simulink model "HQEV_MiL_20160830_integrate_r2017a"  (Simulink 8.9)
settings: Solver=FixedStepDiscrete  StartTime=0.0  StopTime=inf  FixedStep=0.01  RelTol=1e-3  EnableMultiTasking=on
PostLoadFcn:
  | , if any(exist('dsrtsu_mdlpostloadfcn', 'file') == [2, 3, 6]), try dsrtsu_mdlpostloadfcn('Execute', bdroot); catch fprintf('Error in PostLoadFcn (dsrtsu_mdlpostloadfcn) for model "%s":\n %s\n', bdroot, lasterr); end, end,
values from neighbouring files (symbols this model uses):
  Bat_C_Ah = 36    [parameter_V1.mat]
  Bat_ocv_xIndex = [5 10 20 30 40 50 60 70 80 90 95]    [parameter_V1.mat]
  Bat_ocv_z = [329 332 340 345 347 351 358 372 377 386 391]    [parameter_V1.mat]
  Bat_R_ohm_z = [4.41 3.46 1.57 1.07 0.76 0.63 0.55 0.44 0.41 0.4 0.4 3.14 ... (66 elements, 11x6)]    [parameter_V1.mat]
  Bat_SOC_Init = 90    [parameter_V1.mat]
  Env_hum_pct_Ambient = 30    [parameter_V1.mat]
  Env_Slope_deg = 0    [parameter_V1.mat]
  Env_Temp_degC_Ambient = 25    [parameter_V1.mat]
  Env_v_kmph_HWind = 0    [parameter_V1.mat]
  Reducer_F_i = 7.23    [parameter_V1.mat]
  Reducer_R_i = 7.23    [parameter_V1.mat]
  Veh =     [parameter_V1.mat]
  Veh_A_m2_Fr = 2.246    [parameter_V1.mat]
  Veh_F_Brake =     [parameter_V1.mat]
  Veh_fac_AirDrag = 0.326    [parameter_V1.mat]
  Veh_fac_WhDragFrict_0 = 0.011    [parameter_V1.mat]
  Veh_g_mps2_C = 9.81    [parameter_V1.mat]
  Veh_GainBrake =     [parameter_V1.mat]
  Veh_h_m_COGHigh = 0.5    [parameter_V1.mat]
  Veh_J_kgm2_Wh = 1.3635    [parameter_V1.mat]
  Veh_L_m_AxlBas = 2.63    [parameter_V1.mat]
  Veh_M_kg = 1427    [parameter_V1.mat]
  Veh_mu_Brake = 0.4    [parameter_V1.mat]
  Veh_mu_Tyre =     [parameter_V1.mat]
  Veh_num_FrictPair = 8    [parameter_V1.mat]
  Veh_pct_Brk = 70    [parameter_V1.mat]
  Veh_r_dyn =     [parameter_V1.mat]
  Veh_r_m_BrkDisk = 0.136    [parameter_V1.mat]
  Veh_rho_kgpm3_Air = 1.2258    [parameter_V1.mat]
undefined symbols (not defined in the file or in its folder): DiscIntNeverNeededParam, p_bool_False_M, p_bool_True_M
libraries: BaseOperationLib_Browser x38, simulink x8, DTQC_lib x1, ERR_lib x1, MQM_lib x1, PTCL_lib x1, PUD_lib x1, TQD_lib x1, TQR_lib x1, VMM_lib x1, ACCA_lib x1, BBCA_lib x1
(part 7 of 15)

== system HQEV_MiL_20160830_integrate_r2017a/MiL/Test_Integration/MCU_FF/MCU/MCU ==
  In1 : Inport
  Bus Selector : BusSelector  OutputSignals=HCU.HCU_SleepIndication,BMS.BMS_MainPlusContactorCoilState,BMS.BMS_MainMinusContactorCoilState,HCU.HCU_StatusTMRequestToMCU1,HCU.HCU_StopRequestToMCU1,BMS.BMS_PrechargeContactorCoilState,HCU.HCU_RapidDischargeCmdToMCU1,Motor_F.EM1_U,Charger.Charger_OutputVoltage
  Chart : Stateflow chart  TreatAsAtomicUnit=on
  GSD : Subsystem  TreatAsAtomicUnit=on
  Init : Subsystem  TreatAsAtomicUnit=on
  Invalid : Subsystem  TreatAsAtomicUnit=on
  Multiport Switch : MultiPortSwitch  DataPortOrder=Zero-based contiguous  Inputs=9  zeroidx=on
  Precharge : Subsystem  TreatAsAtomicUnit=on
  Rapid_Discharge : Subsystem  TreatAsAtomicUnit=on
  Sleep : Subsystem  TreatAsAtomicUnit=on
  Standby : Subsystem  TreatAsAtomicUnit=on
  Stop : Subsystem  TreatAsAtomicUnit=on
  Torque_Control : Subsystem  TreatAsAtomicUnit=on
  out : Outport
  wires:
  Chart/2(Sleep_Act()) -> [Sleep_Act]
  Chart/3(Init_Act()) -> [Init_Act]
  Chart/4(Precharge_Act()) -> [Precharge_Act]
  Chart/5(Standby_Act()) -> [Standby_Act]
  Chart/6(Torque_Control_Act()) -> [Torque_Control_Act]
  Chart/7(Stop_Act()) -> [Stop_Act]
  Chart/8(GSD_Act()) -> [GSD_Act]
  Chart/9(Rapid_Discharge_Act()) -> [Rapid_Discharge_Act]
  Chart/10(Invalid_Act()) -> [Invalid_Act]
  Chart/1(MCU1_TMStatus) -> [MCU1_TMStatus]
  [Init_Act] -> Init/Trigger
  [Precharge_Act] -> Precharge/Trigger
  [Torque_Control_Act] -> Torque_Control/Trigger
  [Stop_Act] -> Stop/Trigger
  [Rapid_Discharge_Act] -> Rapid_Discharge/Trigger
  [Invalid_Act] -> Invalid/Trigger
  [Standby_Act] -> Standby/Trigger
  [GSD_Act] -> GSD/Trigger
  Init/1(Out1) -> Multiport Switch/2
  Precharge/1(Out1) -> Multiport Switch/3
  Standby/1(Out1) -> Multiport Switch/4
  Torque_Control/1(Out1) -> Multiport Switch/5
  Stop/1(Out1) -> Multiport Switch/6
  GSD/1(Out1) -> Multiport Switch/7
  Rapid_Discharge/1(Out1) -> Multiport Switch/8
  Invalid/1(Out1) -> Multiport Switch/9
  [Sleep_Act] -> Sleep/Trigger
  Sleep/1(Out1) -> Multiport Switch/10
  [MCU1_TMStatus] -> Multiport Switch/1
  In1/1 -> Init/1(In1), Precharge/1(In1), Standby/1(In1), Torque_Control/1(In1), Stop/1(In1), GSD/1(In1), Rapid_Discharge/1(In1), Invalid/1(In1), Sleep/1(In1), Bus Selector/1
  Multiport Switch/1 -> out/1
  Bus Selector/1 -> Chart/1(SleepInd)  "<HCU_SleepIndication>"
  Bus Selector/2 -> Chart/2(BMS_MainPlusContactorState)  "<BMS_MainPlusContactorCoilState>"
  Bus Selector/3 -> Chart/3(BMS_MainMinusContactorCoilState)  "<BMS_MainMinusContactorCoilState>"
  Bus Selector/4 -> Chart/4(HCU_StatusTMRequestToMCU1)  "<HCU_StatusTMRequestToMCU1>"
  Bus Selector/5 -> Chart/5(HCU_StopRequestToMCU1)  "<HCU_StopRequestToMCU1>"
  Bus Selector/6 -> Chart/6(BMS_PrechargeContactorCoilState)  "<BMS_PrechargeContactorCoilState>"
  Bus Selector/7 -> Chart/7(HCU_RapidDischargeCmdToMCU1)  "<HCU_RapidDischargeCmdToMCU1>"
  Bus Selector/8 -> Chart/8(Uc1)  "<EM1_U>"
  Bus Selector/9 -> Chart/9(Charger_OutputVoltage)  "<Charger_OutputVoltage>"

== system HQEV_MiL_20160830_integrate_r2017a/MiL/Test_Integration/MCU_FF/MCU/Signal ==
  bus : Inport
  Bus Creator1 : BusCreator  Inputs=17
  Checksum_MCU1_1 : Subsystem
  Checksum_MCU1_2 : Subsystem
  LiveCounter_MCU1_1 : Subsystem
  LiveCounter_MCU1_2 : Subsystem
  MCU1_ActTMTorque : Subsystem
  MCU1_ActualTMTorqueValid : Subsystem
  MCU1_CalTMTorque : Subsystem
  MCU1_CoolingRequest : Subsystem
  MCU1_PrechargeAllow : Subsystem
  MCU1_ShutdownEnable : Subsystem
  MCU1_TMCapacitanceVoltage : Subsystem
  MCU1_TMErrorStatus : Subsystem
  MCU1_TMSpeed : Subsystem
  MCU1_TMStatus : Subsystem
  MCU1_TM_MAGTorque : Subsystem
  MCU1_TM_MAMTorque : Subsystem
  MCU1_trq_req : Subsystem
  Out1 : Outport
  wires:
  Checksum_MCU1_1/1(out) -> Bus Creator1/1  "Checksum_MCU1_1"
  MCU1_TMSpeed/1(out) -> Bus Creator1/2  "MCU1_TMSpeed"
  MCU1_ActTMTorque/1(out) -> Bus Creator1/3  "MCU1_ActTMTorque"
  LiveCounter_MCU1_1/1(out) -> Bus Creator1/4  "LiveCounter_MCU1_1"
  MCU1_TMCapacitanceVoltage/1(out) -> Bus Creator1/5  "MCU1_TMCapacitanceVoltage"
  MCU1_ActualTMTorqueValid/1(out) -> Bus Creator1/6  "MCU1_ActualTMTorqueValid"
  MCU1_PrechargeAllow/1(out) -> Bus Creator1/7  "MCU1_PrechargeAllow"
  MCU1_TMStatus/1(out) -> Bus Creator1/8  "MCU1_TMStatus"
  MCU1_TMErrorStatus/1(out) -> Bus Creator1/9  "MCU1_TMErrorStatus"
  Checksum_MCU1_2/1(out) -> Bus Creator1/10  "Checksum_MCU1_2"
  MCU1_TM_MAMTorque/1(out) -> Bus Creator1/11  "MCU1_TM_MAMTorque"
  MCU1_TM_MAGTorque/1(out) -> Bus Creator1/12  "MCU1_TM_MAGTorque"
  LiveCounter_MCU1_2/1(out) -> Bus Creator1/13  "LiveCounter_MCU1_2"
  MCU1_CalTMTorque/1(out) -> Bus Creator1/14  "MCU1_CalTMTorque"
  MCU1_CoolingRequest/1(out) -> Bus Creator1/15  "MCU1_CoolingRequest"
  MCU1_trq_req/1(out) -> Bus Creator1/16  "MCU1_trq_req"
  bus/1 -> Checksum_MCU1_1/1(In1), MCU1_TMSpeed/1(In1), MCU1_ActTMTorque/1(In1), LiveCounter_MCU1_1/1(In1), MCU1_TMCapacitanceVoltage/1(In1), MCU1_ActualTMTorqueValid/1(In1), MCU1_PrechargeAllow/1(In1), MCU1_TMStatus/1(In1), MCU1_TMErrorStatus/1(In1), Checksum_MCU1_2/1(In1), MCU1_TM_MAMTorque/1(In1), MCU1_TM_MAGTorque/1(In1), LiveCounter_MCU1_2/1(In1), MCU1_CalTMTorque/1(In1), MCU1_CoolingRequest/1(In1), MCU1_ShutdownEnable/1(In1), MCU1_trq_req/1(In1)
  Bus Creator1/1 -> Out1/1
  MCU1_ShutdownEnable/1(out) -> Bus Creator1/17  "MCU1_ShutdownEnable"

== system HQEV_MiL_20160830_integrate_r2017a/MiL/Test_Integration/MCU_RR/MCU/MCU ==
  In1 : Inport
  Bus Creator : BusCreator  Inputs=14
  Subsystem14 : Subsystem
  Out1 : Outport
  wires:
  In1/1 -> Subsystem14/1(In1)
  Subsystem14/1(MCU2_TMSpeed) -> Bus Creator/1  "MCU2_TMSpeed"
  Subsystem14/2(MCU2_ActTMTorque) -> Bus Creator/2  "MCU2_ActTMTorque"
  Subsystem14/3(MCU2_TMCapacitanceVoltage) -> Bus Creator/3  "MCU2_TMCapacitanceVoltage"
  Subsystem14/4(MCU2_ActualTMTorqueValid) -> Bus Creator/4  "MCU2_ActualTMTorqueValid"
  Subsystem14/5(MCU2_PrechargeAllow) -> Bus Creator/5  "MCU2_PrechargeAllow"
  Subsystem14/6(MCU2_TMStatus) -> Bus Creator/6  "MCU2_TMStatus"
  Subsystem14/7(MCU2_TMErrorStatus) -> Bus Creator/7  "MCU2_TMErrorStatus"
  Subsystem14/8(MCU2_TMMAMTorque) -> Bus Creator/8  "MCU2_TMMAMTorque"
  Subsystem14/9(MCU2_TMMAGTorque) -> Bus Creator/9  "MCU2_TMMAGTorque"
  Subsystem14/10(MCU2_CalTMTorque) -> Bus Creator/10  "MCU2_CalTMTorque"
  Subsystem14/11(MCU2_CoolingRequest) -> Bus Creator/11  "MCU2_CoolingRequest"
  Subsystem14/12(PWM_Status) -> Bus Creator/12  "PWM_Status"
  Subsystem14/13(EM2_trq_req) -> Bus Creator/13  "EM2_trq_Req"
  Bus Creator/1 -> Out1/1
  Subsystem14/14(MCUShutdownEnable) -> Bus Creator/14  "MCUShutdownEnable"

== system HQEV_MiL_20160830_integrate_r2017a/MiL/Test_Integration/MCU_RR/MCU/Signal ==
  in : Inport
  Bus Creator1 : BusCreator  Inputs=17
  Checksum_MCU2_1 : Subsystem
  Checksum_MCU2_2 : Subsystem
  LiveCounter_MCU2_1 : Subsystem
  LiveCounter_MCU2_2 : Subsystem
  MCU2_ActTMTorque : Subsystem
  MCU2_ActualTMTorqueValid : Subsystem
  MCU2_CalTMTorque : Subsystem
  MCU2_CoolingRequest : Subsystem
  MCU2_PrechargeAllow : Subsystem
  MCU2_TMCapacitanceVoltage : Subsystem
  MCU2_TMErrorStatus : Subsystem
  MCU2_TMSpeed : Subsystem
  MCU2_TMStatus : Subsystem
  MCU2_TM_MAGTorque : Subsystem
  MCU2_TM_MAMTorque : Subsystem
  MCU2_trq_req : Subsystem
  MCU2_trq_req1 : Subsystem
  Out1 : Outport
  wires:
  Checksum_MCU2_1/1(out) -> Bus Creator1/1  "Checksum_MCU2_1"
  MCU2_TMSpeed/1(out) -> Bus Creator1/2  "MCU2_TMSpeed"
  MCU2_ActTMTorque/1(out) -> Bus Creator1/3  "MCU2_ActTMTorque"
  LiveCounter_MCU2_1/1(out) -> Bus Creator1/4  "LiveCounter_MCU2_1"
  MCU2_TMCapacitanceVoltage/1(out) -> Bus Creator1/5  "MCU2_TMCapacitanceVoltage"
  MCU2_ActualTMTorqueValid/1(out) -> Bus Creator1/6  "MCU2_ActualTMTorqueValid"
  MCU2_PrechargeAllow/1(out) -> Bus Creator1/7  "MCU2_PrechargeAllow"
  MCU2_TMStatus/1(out) -> Bus Creator1/8  "MCU2_TMStatus"
  MCU2_TMErrorStatus/1(out) -> Bus Creator1/9  "MCU2_TMErrorStatus"
  Checksum_MCU2_2/1(out) -> Bus Creator1/10  "Checksum_MCU2_2"
  MCU2_TM_MAMTorque/1(out) -> Bus Creator1/11  "MCU2_TM_MAMTorque"
  MCU2_TM_MAGTorque/1(out) -> Bus Creator1/12  "MCU2_TM_MAGTorque"
  LiveCounter_MCU2_2/1(out) -> Bus Creator1/13  "LiveCounter_MCU2_2"
  MCU2_CalTMTorque/1(out) -> Bus Creator1/14  "MCU2_CalTMTorque"
  MCU2_CoolingRequest/1(out) -> Bus Creator1/15  "MCU2_CoolingRequest"
  MCU2_trq_req/1(out) -> Bus Creator1/16  "MCU2_trq_req"
  in/1 -> Checksum_MCU2_1/1(In1), MCU2_TMSpeed/1(In1), MCU2_ActTMTorque/1(In1), LiveCounter_MCU2_1/1(In1), MCU2_TMCapacitanceVoltage/1(In1), MCU2_ActualTMTorqueValid/1(In1), MCU2_PrechargeAllow/1(In1), MCU2_TMStatus/1(In1), MCU2_TMErrorStatus/1(In1), Checksum_MCU2_2/1(In1), MCU2_TM_MAMTorque/1(In1), MCU2_TM_MAGTorque/1(In1), LiveCounter_MCU2_2/1(In1), MCU2_CalTMTorque/1(In1), MCU2_CoolingRequest/1(In1), MCU2_trq_req1/1(In1), MCU2_trq_req/1(In1)
  Bus Creator1/1 -> Out1/1
  MCU2_trq_req1/1(out) -> Bus Creator1/17  "MCUShutdownEnable"

== system HQEV_MiL_20160830_integrate_r2017a/MiL/Test_Integration/Motor_FF/Motor/Motor ==
  n_FD_in : Inport
  T_req : Inport  Port=2
  RapidDischargeEnable : Inport  Port=3
  Battery_Voltage : Inport  Port=4
  MainPos_Contactor : Inport  Port=5
  PreCharg_Contactor : Inport  Port=6
  MainNeg_Contactor : Inport  Port=7
  BMS_ChargePlusContactorCoilState : Inport  Port=8
  BMS_ChargeMinusContactorCoilState : Inport  Port=9
  Charger_Status : Inport  Port=10
  Uc_Management : Subsystem
  eMotor : Subsystem
  n_Motor : Outport
  P_Motor_elec : Outport  Port=2
  T_out : Outport  Port=3
  J_out : Outport  Port=4
  P_Motor_loss : Outport  Port=5
  U_TMCap : Outport  Port=6
  wires:
  eMotor/4("J_out ") -> J_out/1
  eMotor/3(EM_trq) -> T_out/1
  eMotor/2(P_Motor_elec) -> P_Motor_elec/1
  eMotor/1(n_Motor) -> n_Motor/1
  eMotor/5(P_Motor_loss) -> P_Motor_loss/1
  Uc_Management/1(Uc) -> U_TMCap/1  "U_TMCap"
  n_FD_in/1 -> eMotor/1(n_FD_in)
  T_req/1 -> eMotor/2(T_req)
  MainPos_Contactor/1 -> Uc_Management/1(MainPos_Contactor)
  PreCharg_Contactor/1 -> Uc_Management/2(PreCharg_Contactor)
  MainNeg_Contactor/1 -> Uc_Management/3(MainNeg_Contactor)
  RapidDischargeEnable/1 -> Uc_Management/4(RapidDischargeEnable)
  Battery_Voltage/1 -> Uc_Management/5(Battery_Voltage)
  BMS_ChargePlusContactorCoilState/1 -> Uc_Management/6(BMS_ChargePlusContactorCoilState)
  BMS_ChargeMinusContactorCoilState/1 -> Uc_Management/7(BMS_ChargeMinusContactorCoilState)
  Charger_Status/1 -> Uc_Management/8(Charger_Status)

== system HQEV_MiL_20160830_integrate_r2017a/MiL/Test_Integration/Motor_RR/Motor/Motor1 ==
  n_FD_in : Inport
  T_req : Inport  Port=2
  RapidDischargeEnable : Inport  Port=3
  Battery_Voltage : Inport  Port=4
  MainPos_Contactor : Inport  Port=5
  PreCharg_Contactor : Inport  Port=6
  MainNeg_Contactor : Inport  Port=7
  BMS_ChargePlusContactorCoilState : Inport  Port=8
  BMS_ChargeMinusContactorCoilState : Inport  Port=9
  Charger_Status : Inport  Port=10
  Uc_Management : Subsystem
  eMotor : Subsystem
  n_Motor : Outport
  P_Motor_elec : Outport  Port=2
  T_out : Outport  Port=3
  J_out : Outport  Port=4
  P_Motor_loss : Outport  Port=5
  U_TMCap : Outport  Port=6
  wires:
  eMotor/4("J_out ") -> J_out/1
  eMotor/3(EM_trq) -> T_out/1
  eMotor/2(P_Motor_elec) -> P_Motor_elec/1
  eMotor/1(n_Motor) -> n_Motor/1
  eMotor/5(P_Motor_loss) -> P_Motor_loss/1
  Uc_Management/1(Uc) -> U_TMCap/1  "U_TMCap"
  n_FD_in/1 -> eMotor/1(n_FD_in)
  T_req/1 -> eMotor/2(T_req)
  MainPos_Contactor/1 -> Uc_Management/1(MainPos_Contactor)
  PreCharg_Contactor/1 -> Uc_Management/2(PreCharg_Contactor)
  MainNeg_Contactor/1 -> Uc_Management/3(MainNeg_Contactor)
  RapidDischargeEnable/1 -> Uc_Management/4(RapidDischargeEnable)
  Battery_Voltage/1 -> Uc_Management/5(Battery_Voltage)
  BMS_ChargePlusContactorCoilState/1 -> Uc_Management/6(BMS_ChargePlusContactorCoilState)
  BMS_ChargeMinusContactorCoilState/1 -> Uc_Management/7(BMS_ChargeMinusContactorCoilState)
  Charger_Status/1 -> Uc_Management/8(Charger_Status)

== system HQEV_MiL_20160830_integrate_r2017a/MiL/Test_Integration/Reducer_F/FinalDrive/FinalDrive ==
  T_in : Inport  Description=Input torque [Nm]
  n_Wheel : Inport  Description=Output speed of final drive [rad/s]  Port=2
  J_in : Inport  Description=Sum of moments of inertia of blocks which are coupled to current block [kg*m^2]  Port=3
  CalcJ_Ratio : Subsystem
  Product1 : Product  RndMeth=Zero
  Subsystem : Subsystem
  Unit Delay : UnitDelay  SampleTime=-1
  Unit Delay1 : UnitDelay  SampleTime=-1
  Unit Delay2 : UnitDelay  InitialCondition=0.01  SampleTime=-1
  ratio : Constant  Value=Reducer_F_i
  "T_out " : Outport  Description=Output torque of final drive [Nm]
  n_in : Outport  Description=Current final drive input speed [rad/s]  Port=2
  "J_out " : Outport  Description=Propagated inertia (input side and current block) [kg*m^2]  Port=3
  wires:
  CalcJ_Ratio/1(J_out [kg*m^2]) -> Unit Delay2/1
  J_in/1 -> CalcJ_Ratio/1(J_pre [kg*m^2])
  Product1/1 -> Unit Delay/1
  Subsystem/1(T_out) -> Unit Delay1/1
  ratio/1 -> Product1/2
  T_in/1 -> Subsystem/1(T_in)
  n_Wheel/1 -> Subsystem/2(n_Wheel), Product1/1
  Unit Delay/1 -> n_in/1
  Unit Delay1/1 -> "T_out "/1
  Unit Delay2/1 -> "J_out "/1

== system HQEV_MiL_20160830_integrate_r2017a/MiL/Test_Integration/Reducer_R/FinalDrive/FinalDrive ==
  T_in : Inport  Description=Input torque [Nm]
  n_Wheel : Inport  Description=Output speed of final drive [rad/s]  Port=2
  J_in [kg*m^2] : Inport  Description=Sum of moments of inertia of blocks which are coupled to current block [kg*m^2]  Port=3
  CalcJ_Ratio : Subsystem
  Constant : Constant  Value=Reducer_R_i
  Product1 : Product  RndMeth=Zero
  Subsystem : Subsystem
  T_out [Nm] : Outport  Description=Output torque of final drive [Nm]
  n_in : Outport  Description=Current final drive input speed [rad/s]  Port=2
  J_out [kg*m^2] : Outport  Description=Propagated inertia (input side and current block) [kg*m^2]  Port=3
  wires:
  n_Wheel/1 -> Product1/1, Subsystem/2(n_Wheel)
  T_in/1 -> Subsystem/1(T_in)
  Constant/1 -> Product1/2
  Subsystem/1(T_out) -> T_out [Nm]/1
  Product1/1 -> n_in/1
  J_in [kg*m^2]/1 -> CalcJ_Ratio/1(J_pre [kg*m^2])
  CalcJ_Ratio/1(J_out [kg*m^2]) -> J_out [kg*m^2]/1

== system HQEV_MiL_20160830_integrate_r2017a/MiL/Test_Integration/Thermal/Thermal/Subsystem ==
  PWM_Pump1 : Inport
  PWM_Pump2 : Inport  Port=2
  pwr_Motor1Loss : Inport  Port=3
  pwr_Motor2Loss : Inport  Port=4
  LowSpdFan_na : Inport  Port=5
  HighSpdFan_na : Inport  Port=6
  pwr_ChargerLoss : Inport  Port=7
  pwr_DCDCLoss : Inport  Port=8
  PWM_BatteryPump : Inport  Port=9
  AC_OnOff : Inport  Port=10
  PWM_PTC : Inport  Port=11
  pwr_BatteryLoss : Inport  Port=12
  BatTempIndex : Inport  Port=13
  Add : Sum
  Battery_Cooling_Circle : Subsystem
  Constant : Constant  Value=0.4
  Constant1 : Constant  Value=0.6
  Motor_Cooling_Circle : Subsystem
  Product : Product  RndMeth=Zero
  Product1 : Product  RndMeth=Zero
  Motor_F_Temp : Outport
  Motor_R_Temp : Outport  Port=2
  DCDC_Temp : Outport  Port=3
  Charger_Temp : Outport  Port=4
  Battery_Temp : Outport  Port=5
  wires:
  pwr_Motor1Loss/1 -> Motor_Cooling_Circle/2(pwr_Motor1Loss)
  pwr_Motor2Loss/1 -> Motor_Cooling_Circle/4(pwr_Motor2Loss)
  PWM_Pump1/1 -> Motor_Cooling_Circle/1(PWM_Pump1)
  PWM_Pump2/1 -> Motor_Cooling_Circle/3(PWM_Pump2)
  pwr_ChargerLoss/1 -> Motor_Cooling_Circle/6(pwr_ChargerLoss)
  pwr_DCDCLoss/1 -> Motor_Cooling_Circle/7(pwr_DCDCLoss)
  Motor_Cooling_Circle/1(Motor_F_Temp) -> Motor_F_Temp/1
  Motor_Cooling_Circle/2(Motor_R_Temp) -> Motor_R_Temp/1
  Motor_Cooling_Circle/4(Charger_Temp) -> Charger_Temp/1
  Motor_Cooling_Circle/3(DCDC_Temp) -> DCDC_Temp/1
  PWM_BatteryPump/1 -> Battery_Cooling_Circle/1(PWM_BatteryPump)
  AC_OnOff/1 -> Battery_Cooling_Circle/2(AC_OnOff)
  PWM_PTC/1 -> Battery_Cooling_Circle/3(PWM_PTC)
  pwr_BatteryLoss/1 -> Battery_Cooling_Circle/4(pwr_BatteryLoss)
  Battery_Cooling_Circle/1(Battery_Temp) -> Battery_Temp/1
  LowSpdFan_na/1 -> Product/1
  HighSpdFan_na/1 -> Product1/1
  Constant/1 -> Product/2
  Constant1/1 -> Product1/2
  Product/1 -> Add/1
  Product1/1 -> Add/2
  Add/1 -> Motor_Cooling_Circle/5(PWM_Fan)
  BatTempIndex/1 -> Battery_Cooling_Circle/5(BatTempIndex)

== system HQEV_MiL_20160830_integrate_r2017a/MiL/Test_Integration/Vehicle/Vehicle/Vehicle ==
  "T_inFront " : Inport  Description=Input torque [Nm]
  "T_inRear " : Inport  Description=Input torque [Nm]  Port=2
  Sig_Brake : Inport  Description=Brake Signal of the driver [%]  Port=3
  v_Hwind_mps : Inport  Description=|  Port=4
      | Current head wind velocity [m/s]
      | >0 Head wind
      | <0 Tail wind
  J_in : Inport  Description=Input inertia [kg*m^2] of previous components  Port=5
  m_add : Inport  Description=Additional vehicle mass which kight be delivered by other components [kg]  Port=6
  Slope_deg : Inport  Description=Current slope of the road [%]  Port=7
  Bus Creator : BusCreator  Inputs=11
  Bus Selector : BusSelector  OutputSignals=v_Hwind,v_Veh,Slope,m_total
  Bus Selector1 : BusSelector  OutputSignals=T_inFront,T_inRear,Sig_Brake,Slope,acc,m_total,Omega_Wh
  Bus Selector2 : BusSelector  OutputSignals=J_in,m_add
  Discrete-Time Integrator : DiscreteIntegrator  SampleTime=-1  ICPrevOutput=DiscIntNeverNeededParam  ICPrevScaledInput=DiscIntNeverNeededParam
  Divide : Product  Inputs=*/
  "J_Equivalent " : Subsystem
  Resistance Torque : Subsystem
  Sum2 : Sum  Inputs=++|
  Unit Delay{,1..3} (4 alike) : UnitDelay  SampleTime=-1
  Wheel Torque : Subsystem
  "[-0.5; +0.5]" : DeadZone  LowerValue=-.5  UpperValue=.5  SaturateOnIntegerOverflow=on
  dw_Correction : Subsystem
  n_Wh : Outport  Description="Current input speed (wheel speed)  in [rad/s]"
  dist [km] : Outport  Description=Run distance of vehicle [m]  Port=2
  v_Veh [km/h] : Outport  Description=Current vehicle speed [km/h]  Port=3
  acc : Outport  Description=Current vehicle speed [km/h]  Port=4
  wires:
  Wheel Torque/1(T_wheel) -> Sum2/2
  Resistance Torque/1(T_Drag [Nm]) -> Sum2/1
  Discrete-Time Integrator/1 -> "[-0.5; +0.5]"/1, Bus Creator/10  "Omega_Wh"
  "[-0.5; +0.5]"/1 -> dw_Correction/2("Omega_out ")
  Sum2/1 -> Divide/1
  Divide/1 -> Discrete-Time Integrator/1, dw_Correction/1(dOmega_out)
  "J_Equivalent "/1(J_Equ) -> Divide/2
  v_Hwind_mps/1 -> Bus Creator/4  "v_Hwind"
  J_in/1 -> Bus Creator/5  "J_in"
  m_add/1 -> Bus Creator/6  "m_add"
  Slope_deg/1 -> Bus Creator/7  "Slope"
  dw_Correction/3(v_Veh [km/h]) -> Bus Creator/8, Unit Delay2/1  "v_Veh"
  Sig_Brake/1 -> Bus Creator/3  "Sig_Brake"
  "T_inFront "/1 -> Bus Creator/1  "T_inFront"
  "T_inRear "/1 -> Bus Creator/2  "T_inRear"
  Bus Selector/1 -> Resistance Torque/1(v_Hwind [m/s])  "<v_Hwind>"
  Bus Selector/2 -> Resistance Torque/2(v_Veh [km/h])  "<v_Veh>"
  Bus Selector/3 -> Resistance Torque/3(phi_Slope [deg])  "<Slope>"
  Bus Selector/4 -> Resistance Torque/4(m_total [kg])  "<m_total>"
  "J_Equivalent "/2(m_total) -> Bus Creator/11  "m_total"
  Bus Selector1/1 -> Wheel Torque/1(T_inFront [Nm])  "<T_inFront>"
  Bus Selector1/2 -> Wheel Torque/2(T_inRear [Nm])  "<T_inRear>"
  Bus Selector1/3 -> Wheel Torque/3(Sig_Brake [%])  "<Sig_Brake>"
  Bus Selector1/4 -> Wheel Torque/4(phi_Slope [deg])  "<Slope>"
  Bus Selector1/5 -> Wheel Torque/5(acc_Veh)  "<acc>"
  Bus Selector1/6 -> Wheel Torque/6(m_total)  "<m_total>"
  Bus Selector1/7 -> Wheel Torque/7(Omega_wh)  "<Omega_Wh>"
  Bus Selector2/1 -> "J_Equivalent "/1(J_in)  "<J_in>"
  Bus Selector2/2 -> "J_Equivalent "/2(m_add [kg])  "<m_add>"
  dw_Correction/4(acc [m/s^2]) -> Bus Creator/9, Unit Delay3/1  "acc"
  dw_Correction/1(dist [km]) -> Unit Delay/1
  dw_Correction/2(n_Wh) -> Unit Delay1/1
  Bus Creator/1 -> Bus Selector/1, Bus Selector1/1, Bus Selector2/1
  Unit Delay/1 -> dist [km]/1
  Unit Delay1/1 -> n_Wh/1
  Unit Delay2/1 -> v_Veh [km/h]/1
  Unit Delay3/1 -> acc/1

== system HQEV_MiL_20160830_integrate_r2017a/MiL/Test_Integration/Accessory/Accessory/Subsystem/vacuum booster ==
  In1 : Inport
  Terminator : Terminator
  kPa : Constant  Value=-600
  vacuum degree : Outport
  wires:
  kPa/1 -> vacuum degree/1
  In1/1 -> Terminator/1

== system HQEV_MiL_20160830_integrate_r2017a/MiL/Test_Integration/BCM/BCM/Check/Subsystem ==
  Constant3 : Constant  Value=0
  Checksum_PSC : Outport
  wires:
  Constant3/1 -> Checksum_PSC/1

== system HQEV_MiL_20160830_integrate_r2017a/MiL/Test_Integration/BCM/BCM/Check/Subsystem1 ==
  Constant4 : Constant  Value=0
  DataBytes : Outport
  wires:
  Constant4/1 -> DataBytes/1

== system HQEV_MiL_20160830_integrate_r2017a/MiL/Test_Integration/BCM/BCM/Check/Subsystem2 ==
  Constant5 : Constant  Value=0
  LiveCounter_PSC : Outport
  wires:
  Constant5/1 -> LiveCounter_PSC/1

== system HQEV_MiL_20160830_integrate_r2017a/MiL/Test_Integration/BCM/BCM/Check/Subsystem3 ==
  Constant6 : Constant  Value=0
  MessageType : Outport
  wires:
  Constant6/1 -> MessageType/1

== system HQEV_MiL_20160830_integrate_r2017a/MiL/Test_Integration/BCM/BCM/Check/Subsystem4 ==
  Constant : Constant  Value=0
  BCM_HighBeamCmd : Outport
  wires:
  Constant/1 -> BCM_HighBeamCmd/1

== system HQEV_MiL_20160830_integrate_r2017a/MiL/Test_Integration/BCM/BCM/Check/Subsystem5 ==
  Constant1 : Constant  Value=0
  DriverDoorSt : Outport
  wires:
  Constant1/1 -> DriverDoorSt/1

== system HQEV_MiL_20160830_integrate_r2017a/MiL/Test_Integration/BCM/BCM/Check/Subsystem6 ==
  Constant2 : Constant  Value=0
  WiperStatus : Outport
  wires:
  Constant2/1 -> WiperStatus/1

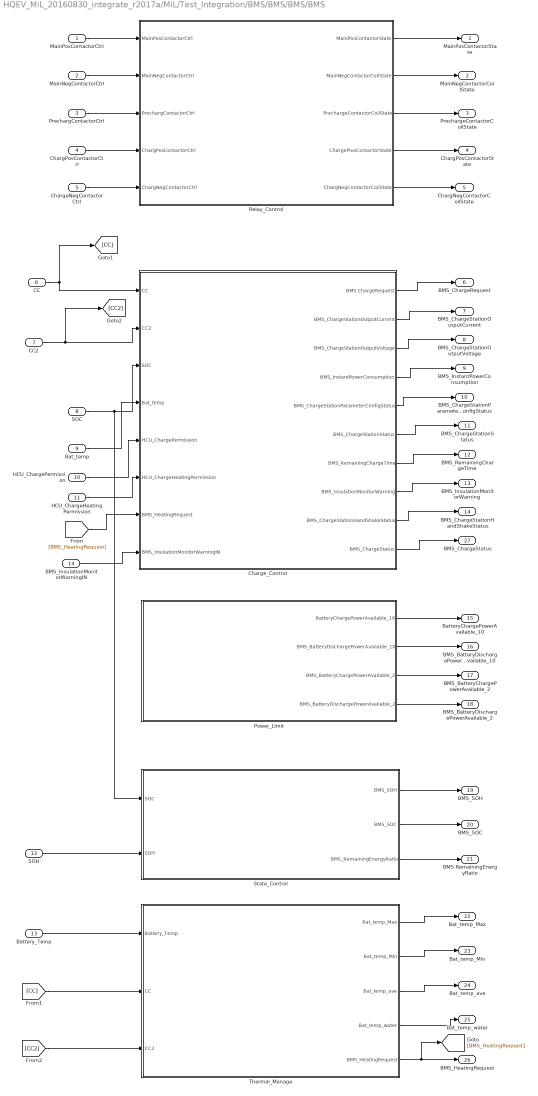
== system HQEV_MiL_20160830_integrate_r2017a/MiL/Test_Integration/BMS/BMS/BMS/BMS ==
  MainPosContactorCtrl : Inport
  MainNegContactorCtrl : Inport  Port=2
  PrechargContactorCtrl : Inport  Port=3
  ChargPosContactorCtrl : Inport  Port=4
  ChargeNegContactorCtrl : Inport  Port=5
  CC : Inport  Port=6
  CC2 : Inport  Port=7
  SOC : Inport  Port=8
  Bat_temp : Inport  Port=9
  HCU_ChargePermission : Inport  Port=10
  HCU_ChargeHeatingPermission : Inport  Port=11
  SOH : Inport  Port=12
  Battery_Temp : Inport  Port=13
  BMS_InsulationMonitorWarningIN : Inport  Port=14
  Charge_Control : Subsystem
  Power_Limit : Subsystem
  Relay_Control : Subsystem
  State_Control : Subsystem
  Thermal_Manage : Subsystem
  MainPosContactorState : Outport
  MainNegContactorCoilState : Outport  Port=2
  PrechargeContactorCoilState : Outport  Port=3
  ChargPosContactorState : Outport  Port=4
  ChargNegContactorCoilState : Outport  Port=5
  BMS_ChargeRequest : Outport  Port=6
  BMS_ChargeStationOutputCurrent : Outport  Port=7
  BMS_ChargeStationOutputVoltage : Outport  Port=8
  BMS_InstantPowerConsumption : Outport  Port=9
  BMS_ChargeStationParameterConfigStatus : Outport  Port=10
  BMS_ChargeStationStatus : Outport  Port=11
  BMS_RemainingChargeTime : Outport  Port=12
  BMS_InsulationMonitorWarning : Outport  Port=13
  BMS_ChargeStationHandShakeStatus : Outport  Port=14
  BatteryChargePowerAvailable_10 : Outport  Port=15
  BMS_BatteryDischargePowerAvailable_10 : Outport  Port=16
  BMS_BatteryChargePowerAvailable_2 : Outport  Port=17
  BMS_BatteryDischargePowerAvailable_2 : Outport  Port=18
  BMS_SOH : Outport  Port=19
  BMS_SOC : Outport  Port=20
  BMS RemainingEnergyRatio : Outport  Port=21
  Bat_temp_Max : Outport  Port=22
  Bat_temp_Min : Outport  Port=23
  Bat_temp_ave : Outport  Port=24
  Bat_temp_water : Outport  Port=25
  BMS_HeatingRequest : Outport  Port=26
  BMS_ChargeStatus : Outport  Port=27
  wires:
  Relay_Control/1(MainPosContactorState) -> MainPosContactorState/1
  Relay_Control/2(MainNegContactorCoilState) -> MainNegContactorCoilState/1
  Relay_Control/3(PrechargeContactorCoilState) -> PrechargeContactorCoilState/1
  Relay_Control/4(ChargePlusContactorState) -> ChargPosContactorState/1
  Relay_Control/5(ChargNegContactorCoilState) -> ChargNegContactorCoilState/1
  Charge_Control/1(BMS ChargeRequest) -> BMS_ChargeRequest/1
  Charge_Control/2(BMS_ChargeStationOutputCurrent) -> BMS_ChargeStationOutputCurrent/1
  Charge_Control/3(BMS_ChargeStationOutputVoltage) -> BMS_ChargeStationOutputVoltage/1
  Charge_Control/4(BMS_InstantPowerConsumption) -> BMS_InstantPowerConsumption/1
  Charge_Control/5(BMS_ChargeStationParameterConfigStatus) -> BMS_ChargeStationParameterConfigStatus/1
  Charge_Control/6(BMS_ChargeStationStatus) -> BMS_ChargeStationStatus/1
  Charge_Control/7(BMS_RemainingChargeTime) -> BMS_RemainingChargeTime/1
  Charge_Control/8(BMS_InsulationMonitorWarning) -> BMS_InsulationMonitorWarning/1
  Charge_Control/9(BMS_ChargeStationHandShakeStatus) -> BMS_ChargeStationHandShakeStatus/1
  Power_Limit/1(BatteryChargePowerAvailable_10) -> BatteryChargePowerAvailable_10/1
  Power_Limit/2(BMS_BatteryDischargePowerAvailable_10) -> BMS_BatteryDischargePowerAvailable_10/1
  Power_Limit/3(BMS_BatteryChargePowerAvailable_2) -> BMS_BatteryChargePowerAvailable_2/1
  Power_Limit/4(BMS_BatteryDischargePowerAvailable_2) -> BMS_BatteryDischargePowerAvailable_2/1
  State_Control/1(BMS_SOH) -> BMS_SOH/1
  State_Control/2(BMS_SOC) -> BMS_SOC/1
  State_Control/3(BMS_RemainingEnergyRatio) -> BMS RemainingEnergyRatio/1
  MainPosContactorCtrl/1 -> Relay_Control/1(MainPosContactorCtrl)
  MainNegContactorCtrl/1 -> Relay_Control/2(MainNegContactorCtrl)
  PrechargContactorCtrl/1 -> Relay_Control/3(PrechargContactorCtrl)
  ChargPosContactorCtrl/1 -> Relay_Control/4(ChargPosContactorCtrl)
  ChargeNegContactorCtrl/1 -> Relay_Control/5(ChargNegContactorCtrl)
  CC/1 -> Charge_Control/1(CC), [CC]
  CC2/1 -> Charge_Control/2(CC2), [CC2]
  SOC/1 -> Charge_Control/3(SOC), State_Control/1(SOC)
  Bat_temp/1 -> Charge_Control/4(Bat_temp)
  HCU_ChargePermission/1 -> Charge_Control/5(HCU_ChargePermission)
  SOH/1 -> State_Control/2(SOH)
  Charge_Control/10(BMS_ChargeStatus) -> BMS_ChargeStatus/1
  Battery_Temp/1 -> Thermal_Manage/1(Battery_Temp)
  HCU_ChargeHeatingPermission/1 -> Charge_Control/6(HCU_ChargeHeatingPermission)
  Thermal_Manage/1(Bat_temp_Max) -> Bat_temp_Max/1
  Thermal_Manage/2(Bat_temp_Min) -> Bat_temp_Min/1
  Thermal_Manage/3(Bat_temp_ave) -> Bat_temp_ave/1
  Thermal_Manage/4(Bat_temp_water) -> Bat_temp_water/1
  Thermal_Manage/5(BMS_HeatingRequest) -> BMS_HeatingRequest/1, [BMS_HeatingRequest]
  [BMS_HeatingRequest] -> Charge_Control/7(BMS_HeatingRequest)
  [CC] -> Thermal_Manage/2(CC)
  [CC2] -> Thermal_Manage/3(CC2)
  BMS_InsulationMonitorWarningIN/1 -> Charge_Control/8(BMS_InsulationMonitorWarningIN)

== system HQEV_MiL_20160830_integrate_r2017a/MiL/Test_Integration/BMS/BMS/Signal/BMS_BatteryChargePowerAvailable_10 ==
  In1 : Inport
  Bus Selector : BusSelector  OutputSignals=BMS.BatteryChargePowerAvailable_10
  out : Outport
  wires:
  In1/1 -> Bus Selector/1
  Bus Selector/1 -> out/1  "<BatteryChargePowerAvailable_10>"

== system HQEV_MiL_20160830_integrate_r2017a/MiL/Test_Integration/BMS/BMS/Signal/BMS_BatteryChargePowerAvailable_2 ==
  In : Inport
  Bus Selector : BusSelector  OutputSignals=BMS.BMS_BatteryChargePowerAvailable_2
  out : Outport
  wires:
  Bus Selector/1 -> out/1  "<BMS_BatteryChargePowerAvailable_2>"
  In/1 -> Bus Selector/1

== system HQEV_MiL_20160830_integrate_r2017a/MiL/Test_Integration/BMS/BMS/Signal/BMS_BatteryDischargePowerAvailable_10 ==
  In1 : Inport
  Bus Selector : BusSelector  OutputSignals=BMS.BMS_BatteryDischargePowerAvailable_10
  out : Outport
  wires:
  Bus Selector/1 -> out/1  "<BMS_BatteryDischargePowerAvailable_10>"
  In1/1 -> Bus Selector/1

== system HQEV_MiL_20160830_integrate_r2017a/MiL/Test_Integration/BMS/BMS/Signal/BMS_BatteryDischargePowerAvailable_2 ==
  In1 : Inport
  Bus Selector : BusSelector  OutputSignals=BMS.BMS_BatteryDischargePowerAvailable_2
  out : Outport
  wires:
  In1/1 -> Bus Selector/1
  Bus Selector/1 -> out/1  "<BMS_BatteryDischargePowerAvailable_2>"

== system HQEV_MiL_20160830_integrate_r2017a/MiL/Test_Integration/BMS/BMS/Signal/BMS_BatteryPackCurrent ==
  In1 : Inport
  Bus Selector : BusSelector  OutputSignals=signal1.Battery.Battery_Current
  out : Outport
  wires:
  In1/1 -> Bus Selector/1
  Bus Selector/1 -> out/1  "<Battery_Current>"

== system HQEV_MiL_20160830_integrate_r2017a/MiL/Test_Integration/BMS/BMS/Signal/BMS_BatteryPackInletWaterTemperature ==
  In1 : Inport
  Bus Selector : BusSelector  OutputSignals=BMS.Bat_temp_water
  out : Outport
  wires:
  In1/1 -> Bus Selector/1
  Bus Selector/1 -> out/1  "<Bat_temp_water>"

== system HQEV_MiL_20160830_integrate_r2017a/MiL/Test_Integration/BMS/BMS/Signal/BMS_BatteryPackMAXTemperature ==
  In1 : Inport
  Bus Selector : BusSelector  OutputSignals=BMS.Bat_temp_Max
  out : Outport
  wires:
  Bus Selector/1 -> out/1  "<Bat_temp_Max>"
  In1/1 -> Bus Selector/1

== system HQEV_MiL_20160830_integrate_r2017a/MiL/Test_Integration/BMS/BMS/Signal/BMS_BatteryPackMINTemperature ==
  In1 : Inport
  Bus Selector : BusSelector  OutputSignals=BMS.Bat_temp_Min
  out : Outport
  wires:
  In1/1 -> Bus Selector/1
  Bus Selector/1 -> out/1  "<Bat_temp_Min>"

== system HQEV_MiL_20160830_integrate_r2017a/MiL/Test_Integration/BMS/BMS/Signal/BMS_BatteryPackSOC ==
  In1 : Inport
  Bus Selector : BusSelector  OutputSignals=BMS.BMS_SOC
  out : Outport
  wires:
  In1/1 -> Bus Selector/1
  Bus Selector/1 -> out/1  "<BMS_SOC>"

== system HQEV_MiL_20160830_integrate_r2017a/MiL/Test_Integration/BMS/BMS/Signal/BMS_BatteryPackSOH ==
  In1 : Inport
  Bus Selector : BusSelector  OutputSignals=BMS.BMS_SOH
  out : Outport
  wires:
  In1/1 -> Bus Selector/1
  Bus Selector/1 -> out/1  "<BMS_SOH>"

== system HQEV_MiL_20160830_integrate_r2017a/MiL/Test_Integration/BMS/BMS/Signal/BMS_BatteryPackStatus ==
  In1 : Inport
  Bus Selector : BusSelector  OutputSignals=signal1.IO.BMS_BatteryPackStatus
  BMS_BatteryPackStatus : Outport
  wires:
  In1/1 -> Bus Selector/1
  Bus Selector/1 -> BMS_BatteryPackStatus/1  "<BMS_BatteryPackStatus>"

== system HQEV_MiL_20160830_integrate_r2017a/MiL/Test_Integration/BMS/BMS/Signal/BMS_BatteryPackTemperature ==
  In1 : Inport
  Bus Selector : BusSelector  OutputSignals=BMS.Bat_temp_ave
  out : Outport
  wires:
  In1/1 -> Bus Selector/1
  Bus Selector/1 -> out/1  "<Bat_temp_ave>"

== system HQEV_MiL_20160830_integrate_r2017a/MiL/Test_Integration/BMS/BMS/Signal/BMS_BatteryPackVoltage ==
  In1 : Inport
  Bus Selector : BusSelector  OutputSignals=signal1.Battery.Battery_Voltage
  out : Outport
  wires:
  In1/1 -> Bus Selector/1
  Bus Selector/1 -> out/1  "<Battery_Voltage>"

== system HQEV_MiL_20160830_integrate_r2017a/MiL/Test_Integration/BMS/BMS/Signal/BMS_ChargeMinusContactorCoilFault ==
  In1 : Inport
  Constant1 : Constant  Value=0
  Terminator : Terminator
  out : Outport
  wires:
  In1/1 -> Terminator/1
  Constant1/1 -> out/1

== system HQEV_MiL_20160830_integrate_r2017a/MiL/Test_Integration/BMS/BMS/Signal/BMS_ChargeMinusContactorCoilState ==
  In1 : Inport
  Bus Selector : BusSelector  OutputSignals=BMS.ChargeMinusContactorCoilState
  out : Outport
  wires:
  Bus Selector/1 -> out/1  "<ChargeMinusContactorCoilState>"
  In1/1 -> Bus Selector/1

== system HQEV_MiL_20160830_integrate_r2017a/MiL/Test_Integration/BMS/BMS/Signal/BMS_ChargePlusContactorCoilFault ==
  In1 : Inport
  Constant1 : Constant  Value=0
  Terminator : Terminator
  out : Outport
  wires:
  In1/1 -> Terminator/1
  Constant1/1 -> out/1

== system HQEV_MiL_20160830_integrate_r2017a/MiL/Test_Integration/BMS/BMS/Signal/BMS_ChargePlusContactorCoilState ==
  In1 : Inport
  Bus Selector : BusSelector  OutputSignals=BMS.ChargePlusContactorState
  out : Outport
  wires:
  Bus Selector/1 -> out/1  "<ChargePlusContactorState>"
  In1/1 -> Bus Selector/1

== system HQEV_MiL_20160830_integrate_r2017a/MiL/Test_Integration/BMS/BMS/Signal/BMS_ChargePlusContactorFault ==
  In1 : Inport
  Constant : Constant  Value=0
  Terminator : Terminator
  out : Outport
  wires:
  In1/1 -> Terminator/1
  Constant/1 -> out/1

== system HQEV_MiL_20160830_integrate_r2017a/MiL/Test_Integration/BMS/BMS/Signal/BMS_ChargeRequest ==
  In1 : Inport
  Bus Selector : BusSelector  OutputSignals=BMS.BMS_ChargeRequest
  out : Outport
  wires:
  In1/1 -> Bus Selector/1
  Bus Selector/1 -> out/1  "<BMS_ChargeRequest>"

== system HQEV_MiL_20160830_integrate_r2017a/MiL/Test_Integration/BMS/BMS/Signal/BMS_ChargeStationHandShakeStatus ==
  In1 : Inport
  Bus Selector : BusSelector  OutputSignals=BMS.BMS_ChargeStationHandShakeStatus
  out : Outport
  wires:
  In1/1 -> Bus Selector/1
  Bus Selector/1 -> out/1  "<BMS_ChargeStationHandShakeStatus>"

== system HQEV_MiL_20160830_integrate_r2017a/MiL/Test_Integration/BMS/BMS/Signal/BMS_ChargeStationOutputCurrent ==
  In1 : Inport
  Bus Selector : BusSelector  OutputSignals=BMS.BMS_ChargeStationOutputCurrent
  out : Outport
  wires:
  Bus Selector/1 -> out/1  "<BMS_ChargeStationOutputCurrent>"
  In1/1 -> Bus Selector/1

== system HQEV_MiL_20160830_integrate_r2017a/MiL/Test_Integration/BMS/BMS/Signal/BMS_ChargeStationOutputVoltage ==
  In1 : Inport
  Bus Selector : BusSelector  OutputSignals=BMS.BMS_ChargeStationOutputVoltage
  out : Outport
  wires:
  Bus Selector/1 -> out/1  "<BMS_ChargeStationOutputVoltage>"
  In1/1 -> Bus Selector/1

== system HQEV_MiL_20160830_integrate_r2017a/MiL/Test_Integration/BMS/BMS/Signal/BMS_ChargeStationParameterConfigStatus ==
  In1 : Inport
  Bus Selector : BusSelector  OutputSignals=BMS.BMS_ChargeStationParameterConfigStatus
  out : Outport
  wires:
  In1/1 -> Bus Selector/1
  Bus Selector/1 -> out/1  "<BMS_ChargeStationParameterConfigStatus>"

== system HQEV_MiL_20160830_integrate_r2017a/MiL/Test_Integration/BMS/BMS/Signal/BMS_ChargeStationStatus ==
  In1 : Inport
  Bus Selector : BusSelector  OutputSignals=BMS.BMS_ChargeStationStatus
  out : Outport
  wires:
  In1/1 -> Bus Selector/1
  Bus Selector/1 -> out/1  "<BMS_ChargeStationStatus>"

== system HQEV_MiL_20160830_integrate_r2017a/MiL/Test_Integration/BMS/BMS/Signal/BMS_ChargeStatus ==
  In1 : Inport
  Bus Selector : BusSelector  OutputSignals=BMS.BMS_ChargeStatus
  out : Outport
  wires:
  In1/1 -> Bus Selector/1
  Bus Selector/1 -> out/1  "<BMS_ChargeStatus>"

== system HQEV_MiL_20160830_integrate_r2017a/MiL/Test_Integration/BMS/BMS/Signal/BMS_FaultDisposeSignal ==
  In1 : Inport
  Constant : Constant  Value=0
  Terminator : Terminator
  out : Outport
  wires:
  Constant/1 -> out/1
  In1/1 -> Terminator/1

== system HQEV_MiL_20160830_integrate_r2017a/MiL/Test_Integration/BMS/BMS/Signal/BMS_HeatingRequest ==
  In1 : Inport
  Bus Selector : BusSelector  OutputSignals=BMS.BMS_HeatingRequest
  out : Outport
  wires:
  In1/1 -> Bus Selector/1
  Bus Selector/1 -> out/1  "<BMS_HeatingRequest>"

== system HQEV_MiL_20160830_integrate_r2017a/MiL/Test_Integration/BMS/BMS/Signal/BMS_InstantPowerConsumption ==
  In1 : Inport
  Constant : Constant  Value=0
  Terminator : Terminator
  out : Outport
  wires:
  Constant/1 -> out/1
  In1/1 -> Terminator/1

== system HQEV_MiL_20160830_integrate_r2017a/MiL/Test_Integration/BMS/BMS/Signal/BMS_InsulationMonitorWarning ==
  In1 : Inport
  Bus Selector : BusSelector  OutputSignals=BMS.BMS_InsulationMonitorWarning
  out : Outport
  wires:
  In1/1 -> Bus Selector/1
  Bus Selector/1 -> out/1  "<BMS_InsulationMonitorWarning>"

== system HQEV_MiL_20160830_integrate_r2017a/MiL/Test_Integration/BMS/BMS/Signal/BMS_MainMinusContactorCoilFault ==
  In1 : Inport
  Constant : Constant  Value=0
  Terminator : Terminator
  out : Outport
  wires:
  In1/1 -> Terminator/1
  Constant/1 -> out/1

== system HQEV_MiL_20160830_integrate_r2017a/MiL/Test_Integration/BMS/BMS/Signal/BMS_MainMinusContactorCoilState ==
  In1 : Inport
  Bus Selector : BusSelector  OutputSignals=BMS.MainMinusContactorCoilState
  out : Outport
  wires:
  Bus Selector/1 -> out/1  "<MainMinusContactorCoilState>"
  In1/1 -> Bus Selector/1

== system HQEV_MiL_20160830_integrate_r2017a/MiL/Test_Integration/BMS/BMS/Signal/BMS_MainPlusContactorCoilFault ==
  In1 : Inport
  Constant : Constant  Value=0
  Terminator : Terminator
  out : Outport
  wires:
  In1/1 -> Terminator/1
  Constant/1 -> out/1

== system HQEV_MiL_20160830_integrate_r2017a/MiL/Test_Integration/BMS/BMS/Signal/BMS_MainPlusContactorCoilState ==
  In1 : Inport
  Bus Selector : BusSelector  OutputSignals=BMS.MainPlusContactorState
  out : Outport
  wires:
  Bus Selector/1 -> out/1  "<MainPlusContactorState>"
  In1/1 -> Bus Selector/1

== system HQEV_MiL_20160830_integrate_r2017a/MiL/Test_Integration/BMS/BMS/Signal/BMS_MainPlusContactorFault ==
  In1 : Inport
  Constant : Constant  Value=0
  Terminator : Terminator
  out : Outport
  wires:
  Constant/1 -> out/1
  In1/1 -> Terminator/1

== system HQEV_MiL_20160830_integrate_r2017a/MiL/Test_Integration/BMS/BMS/Signal/BMS_PrechargeContactorCoilFault ==
  In1 : Inport
  Constant1 : Constant  Value=0
  Terminator : Terminator
  out : Outport
  wires:
  In1/1 -> Terminator/1
  Constant1/1 -> out/1

== system HQEV_MiL_20160830_integrate_r2017a/MiL/Test_Integration/BMS/BMS/Signal/BMS_PrechargeContactorCoilState ==
  In1 : Inport
  Bus Selector : BusSelector  OutputSignals=BMS.PrechargeContactorCoilState
  out : Outport
  wires:
  Bus Selector/1 -> out/1  "<PrechargeContactorCoilState>"
  In1/1 -> Bus Selector/1

== system HQEV_MiL_20160830_integrate_r2017a/MiL/Test_Integration/BMS/BMS/Signal/BMS_RemainingChargeTime ==
  In1 : Inport
  Constant : Constant  Value=50
  Terminator : Terminator
  out : Outport
  wires:
  Constant/1 -> out/1
  In1/1 -> Terminator/1

== system HQEV_MiL_20160830_integrate_r2017a/MiL/Test_Integration/BMS/BMS/Signal/BMS_RemainingEnergyRatio ==
  In1 : Inport
  Bus Selector : BusSelector  OutputSignals=BMS.BMS RemainingEnergyRatio
  out : Outport
  wires:
  In1/1 -> Bus Selector/1
  Bus Selector/1 -> out/1  "<BMS RemainingEnergyRatio>"

== system HQEV_MiL_20160830_integrate_r2017a/MiL/Test_Integration/BMS/BMS/Signal/Checksum_BMS_1 ==
  In1 : Inport
  Constant : Constant  Value=0
  Terminator : Terminator
  out : Outport
  wires:
  Constant/1 -> out/1
  In1/1 -> Terminator/1

== system HQEV_MiL_20160830_integrate_r2017a/MiL/Test_Integration/BMS/BMS/Signal/Checksum_BMS_2 ==
  In1 : Inport
  Terminator : Terminator
  kW : Constant  Value=100
  Checksum_BMS_2 : Outport
  wires:
  In1/1 -> Terminator/1
  kW/1 -> Checksum_BMS_2/1

== system HQEV_MiL_20160830_integrate_r2017a/MiL/Test_Integration/BMS/BMS/Signal/Checksum_BMS_3 ==
  In1 : Inport
  Constant : Constant  Value=0
  Terminator : Terminator
  out : Outport
  wires:
  In1/1 -> Terminator/1
  Constant/1 -> out/1

== system HQEV_MiL_20160830_integrate_r2017a/MiL/Test_Integration/BMS/BMS/Signal/Checksum_BMS_6 ==
  In1 : Inport
  Constant : Constant  Value=0
  Terminator : Terminator
  out : Outport
  wires:
  Constant/1 -> out/1
  In1/1 -> Terminator/1

== system HQEV_MiL_20160830_integrate_r2017a/MiL/Test_Integration/BMS/BMS/Signal/LiveCounter_BMS_1 ==
  In1 : Inport
  Constant : Constant  Value=0
  Terminator : Terminator
  out : Outport
  wires:
  Constant/1 -> out/1
  In1/1 -> Terminator/1

== system HQEV_MiL_20160830_integrate_r2017a/MiL/Test_Integration/BMS/BMS/Signal/LiveCounter_BMS_2 ==
  In1 : Inport
  Terminator : Terminator
  kW : Constant  Value=0
  out : Outport
  wires:
  In1/1 -> Terminator/1
  kW/1 -> out/1

== system HQEV_MiL_20160830_integrate_r2017a/MiL/Test_Integration/BMS/BMS/Signal/LiveCounter_BMS_3 ==
  In1 : Inport
  Constant : Constant  Value=0
  Terminator : Terminator
  out : Outport
  wires:
  Constant/1 -> out/1
  In1/1 -> Terminator/1

== system HQEV_MiL_20160830_integrate_r2017a/MiL/Test_Integration/BMS/BMS/Signal/LiveCounter_BMS_6 ==
  In1 : Inport
  Constant : Constant  Value=0
  Terminator : Terminator
  out : Outport
  wires:
  In1/1 -> Terminator/1
  Constant/1 -> out/1

== system HQEV_MiL_20160830_integrate_r2017a/MiL/Test_Integration/Battery/Battery/Battery/Battery_Output ==
  note: Positive for Discharge
  Bat_pwr_out : Inport
  Battery_Temp : Inport  Port=2
  SOC : Inport  Port=3
  Battery_characteristic : Subsystem
  Subsystem : Subsystem
  Battery_Voltage : Outport
  Battery_Power_loss : Outport  Port=2
  Battery_Current : Outport  Port=3
  wires:
  Battery_characteristic/1(OCV) -> Subsystem/1(OCV)
  Battery_characteristic/2(ohm) -> Subsystem/2(Internal_Resistance)
  SOC/1 -> Battery_characteristic/1(SOC)
  Subsystem/1(Bat_Voltage) -> Battery_Voltage/1
  Subsystem/2(Bat_Current) -> Battery_Current/1
  Bat_pwr_out/1 -> Subsystem/3(Bat_pwr_out)
  Battery_Temp/1 -> Battery_characteristic/2(Battery_Temp)
  Subsystem/3(Bat_pwr_loss) -> Battery_Power_loss/1

== system HQEV_MiL_20160830_integrate_r2017a/MiL/Test_Integration/Battery/Battery/Battery/SOC_Subsystem ==
  note: SOC=Remaining_Capacity/Full_Capacity
  Battery_Current : Inport
  SOCIndex : Inport  Port=2
  Ah : Product  Inputs=*/
  Ah1 : Product  Inputs=*/
  As : DiscreteIntegrator  SampleTime=-1  ICPrevOutput=DiscIntNeverNeededParam  ICPrevScaledInput=DiscIntNeverNeededParam
  Capacity_Ah : Constant  Value=Bat_C_Ah
  Capacity_Ah1 : Constant  Value=Bat_C_Ah
  Compare To Constant : simulink/Logic and Bit Operations/Compare To Constant  relop===  const=0  OutDataTypeStr=boolean
  Constant : Constant  Value=100
  Constant1 : Constant  Value=3600
  Constant2 : Constant  Value=100
  I1 : Product  Inputs=*/
  Product : Product  RndMeth=Zero
  Product1 : Product  RndMeth=Zero
  SOC0 : Constant  Value=Bat_SOC_Init
  Subtract : Sum  Inputs=+-
  Switch : Switch  Criteria=u2 > Threshold
  Unit Delay : UnitDelay  SampleTime=-1
  SOC : Outport
  wires:
  As/1 -> Ah/1
  Capacity_Ah/1 -> I1/2
  Subtract/1 -> I1/1
  Product1/1 -> SOC/1
  Ah1/1 -> Product/1
  Battery_Current/1 -> Unit Delay/1
  Unit Delay/1 -> As/1
  Capacity_Ah1/1 -> Product/2
  Product/1 -> Subtract/1
  Ah/1 -> Subtract/2
  I1/1 -> Product1/1
  Constant/1 -> Product1/2
  Constant1/1 -> Ah/2
  Constant2/1 -> Ah1/2
  SOCIndex/1 -> Switch/3, Compare To Constant/1
  Compare To Constant/1 -> Switch/2
  SOC0/1 -> Switch/1
  Switch/1 -> Ah1/1

== system HQEV_MiL_20160830_integrate_r2017a/MiL/Test_Integration/Battery/Battery/Battery/Subsystem ==
  EM1_pwr_elec : Inport
  EM2_pwr_elec : Inport  Port=2
  DCDC_pwr_in : Inport  Port=3
  AC_pwr_elec : Inport  Port=4
  Charger_OutputVoltage : Inport  Port=5
  Charger_OutputCurrent : Inport  Port=6
  HCU_ChargerPermission : Inport  Port=7
  Add{1..4} (4 alike) : Sum
  Data Type Conversion : DataTypeConversion
  Product : Product  RndMeth=Zero
  Product1 : Product  RndMeth=Zero
  Bat_pwr_out : Outport
  wires:
  Add1/1 -> Add2/1
  EM1_pwr_elec/1 -> Add1/1
  EM2_pwr_elec/1 -> Add1/2
  DCDC_pwr_in/1 -> Add2/2
  Add2/1 -> Add3/1
  Add3/1 -> Add4/1
  Add4/1 -> Bat_pwr_out/1
  AC_pwr_elec/1 -> Add3/2
  Charger_OutputVoltage/1 -> Product/1
  Charger_OutputCurrent/1 -> Product/2
  HCU_ChargerPermission/1 -> Data Type Conversion/1
  Product/1 -> Product1/1
  Product1/1 -> Add4/2
  Data Type Conversion/1 -> Product1/2

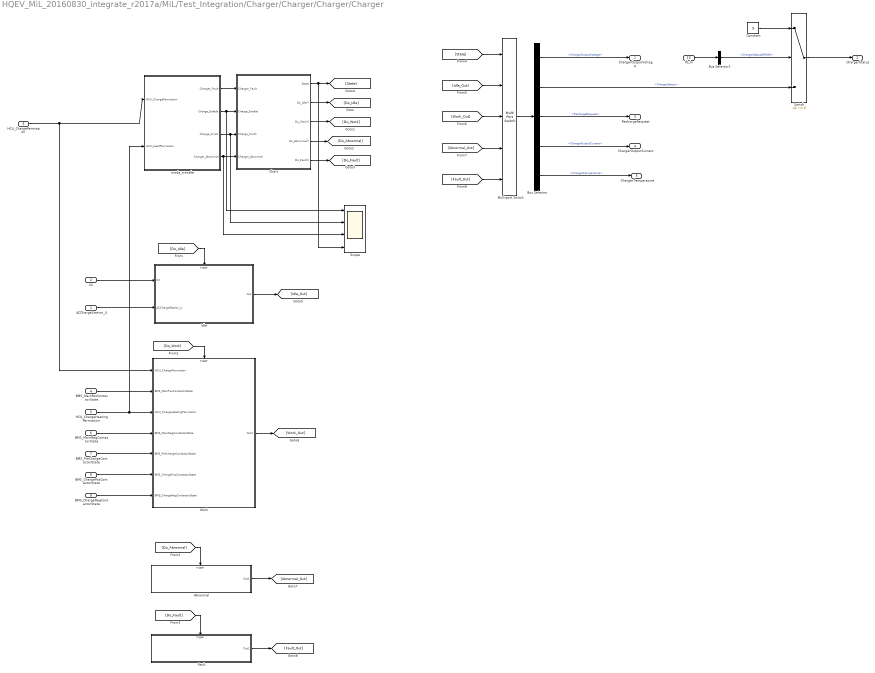
== system HQEV_MiL_20160830_integrate_r2017a/MiL/Test_Integration/Charger/Charger/Charger/Charger ==
  ACChargeStation_U : Inport
  CC : Inport  Port=2
  HCU_ChargePermission : Inport  Port=3
  BMS_MainPosContactorState : Inport  Port=4
  HCU_ChargeHeatingPermission : Inport  Port=5
  BMS_MainNegContactorState : Inport  Port=6
  BMS_PreChargeContactorState : Inport  Port=7
  BMS_ChargePosContactorState : Inport  Port=8
  BMS_ChargeNegContactorState : Inport  Port=9
  IO_In : Inport  Port=10
  Abnormal : Subsystem  TreatAsAtomicUnit=on
  Bus Selector : BusSelector  OutputSignals=ChargerOutputVoltage,ChargerStatus,RechargeRequest,ChargerOutputCurrent,ChargerTemperature
  Bus Selector1 : BusSelector  OutputSignals=IO.ChargerStatusERROR
  Chart : Stateflow chart  TreatAsAtomicUnit=on
  Constant : Constant  Value=3
  Fault : Subsystem  TreatAsAtomicUnit=on
  Idle : Subsystem  TreatAsAtomicUnit=on
  Multiport Switch : MultiPortSwitch  Inputs=4
  Scope : Scope  NumInputPorts=4
  Switch : Switch  Criteria=u2 ~= 0
  Work : Subsystem  TreatAsAtomicUnit=on
  mode_transfer : Subsystem
  ChargerOutputVoltage : Outport
  ChargerStatus : Outport  Port=2
  RechargeRequest : Outport  Port=3
  ChargerOutputCurrent : Outport  Port=4
  ChargerTemperature : Outport  Port=5
  wires:
  [State] -> Multiport Switch/1
  mode_transfer/1(Charger_Fault) -> Chart/1(Charger_Fault)
  mode_transfer/2(Charge_Enable) -> Chart/2(Charge_Enable), Scope/1
  mode_transfer/3(Charge_Finish) -> Chart/3(Charge_Finish), Scope/2
  mode_transfer/4(Charger_Abnormal) -> Chart/4(Charger_Abnormal), Scope/3
  Chart/2(Do_Idle()) -> [Do_Idle]
  Chart/3(Do_Work()) -> [Do_Work]
  Chart/4(Do_Abnormal()) -> [Do_Abnormal]
  Chart/5(Do_Fault()) -> [Do_Fault]
  [Do_Idle] -> Idle/Trigger
  [Do_Work] -> Work/Trigger
  [Do_Abnormal] -> Abnormal/Trigger
  [Do_Fault] -> Fault/Trigger
  Chart/1(State) -> [State], Scope/4
  Multiport Switch/1 -> Bus Selector/1
  Bus Selector/1 -> ChargerOutputVoltage/1  "<ChargerOutputVoltage>"
  Bus Selector/3 -> RechargeRequest/1  "<RechargeRequest>"
  Bus Selector/4 -> ChargerOutputCurrent/1  "<ChargerOutputCurrent>"
  Bus Selector/5 -> ChargerTemperature/1  "<ChargerTemperature>"
  HCU_ChargePermission/1 -> mode_transfer/1(HCU_ChargePermission), Work/1(HCU_ChargePermission)
  CC/1 -> Idle/1(CC)
  ACChargeStation_U/1 -> Idle/2(ACChargeStation_U)
  Idle/1(Out) -> [Idle_Out]
  Work/1(Out1) -> [Work_Out]
  Abnormal/1(Out1) -> [Abnormal_Out]
  Fault/1(Out1) -> [Fault_Out]
  BMS_MainPosContactorState/1 -> Work/2(BMS_MainPosContactorState)
  HCU_ChargeHeatingPermission/1 -> Work/3(HCU_ChargeHeatingPermission), mode_transfer/2(HCU_HeatPermission)
  BMS_MainNegContactorState/1 -> Work/4(BMS_MainNegContactorState)
  BMS_PreChargeContactorState/1 -> Work/5(BMS_PreChargeContactorState)
  BMS_ChargePosContactorState/1 -> Work/6(BMS_ChargePosContactorState)
  BMS_ChargeNegContactorState/1 -> Work/7(BMS_ChargeNegContactorState)
  [Idle_Out] -> Multiport Switch/2
  [Work_Out] -> Multiport Switch/3
  [Abnormal_Out] -> Multiport Switch/4
  [Fault_Out] -> Multiport Switch/5
  IO_In/1 -> Bus Selector1/1
  Bus Selector1/1 -> Switch/2  "<ChargerStatusERROR>"
  Bus Selector/2 -> Switch/3  "<ChargerStatus>"
  Switch/1 -> ChargerStatus/1
  Constant/1 -> Switch/1

== system HQEV_MiL_20160830_integrate_r2017a/MiL/Test_Integration/Cycle/Cycle/Cycle/SimTimeControl ==
  RunSignal : Inport
  Constant1 : Constant  Value=1180
  Constant5 : Constant
  Constant6 : Constant  Value=0
  Discrete-Time Integrator : DiscreteIntegrator  ExternalReset=rising  SampleTime=0.01  ICPrevOutput=DiscIntNeverNeededParam  ICPrevScaledInput=DiscIntNeverNeededParam
  Relational Operator : RelationalOperator  OutDataTypeStr=boolean  RndMeth=Nearest
  Switch : Switch  Criteria=u2 > Threshold  Threshold=0.5
  Unit Delay : UnitDelay  SampleTime=0.01
  time : Outport
  wires:
  Constant5/1 -> Switch/1
  Constant6/1 -> Switch/3
  Switch/1 -> Discrete-Time Integrator/1
  Discrete-Time Integrator/1 -> time/1, Relational Operator/1
  Constant1/1 -> Relational Operator/2
  Relational Operator/1 -> Unit Delay/1
  RunSignal/1 -> Switch/2
  Unit Delay/1 -> Discrete-Time Integrator/2
